simulink model "Napdangdi"  (R2016a)
settings: Solver=FixedStepAuto  StartTime=0.0  StopTime=inf  FixedStep=0.04  RelTol=1e-3
InitFcn:
  | ts=0.04;
  | 
  | v = evalin('base', 'deta1');
  | Deta1 = v;
  | v = evalin('base', 'deta2');
  | Deta2 = v;
  | v = evalin('base', 'deta3');
  | Deta3 = v;
  | v = evalin('base', 'deta5');
  | Deta5 = v;
  | v = evalin('base', 'deta6');
  | Deta6 = v;
  | v = evalin('base', 'deta7');
  | Deta7 = v;
  | v = evalin('base', 'deta8');
  | Deta8 = v;
  | v = evalin('base', 'deta10');
  | Deta10 = v;
  | v = evalin('base', 'deta11');
  | Deta11 = v;
  | v = evalin('base', 'deta12');
  | Deta12 = v;
values from neighbouring files (symbols this model uses):
  deta1 = atan(l.y./l.z)    [biped_backward.m]    (also in dang1.mat = [-0.00346399618455 -0.00193508096073 0.00231722618874 0.0086; dang3.mat = [-0.00346399618455 -0.00185781856517 0.00257715248671 0.0091; dang4.mat = [-0.00346399618455 -0.000867212023118 0.00606051163541 0.015; inverse_kinematic.m = atan(y_l/z_l))
  deta10 = pi-detaC    [biped_backward.m]    (also in inverse_kinematic.m; inverse_kinematics.m)
  deta11 = (deta10-deta8)    [biped_backward.m]    (also in inverse_kinematic.m = (deta10 - deta8); inverse_kinematics.m = deta10-deta8)
  deta12 = atan(r.y./r.z)    [biped_backward.m]    (also in inverse_kinematic.m = atan(y_r/z_r); inverse_kinematics.m)
  deta2 = (deta3-deta5)    [biped_backward.m]    (also in inverse_kinematic.m = (deta3 - deta5); inverse_kinematics.m)
  deta3 = pi-detaA    [biped_backward.m]    (also in inverse_kinematic.m; inverse_kinematics.m)
  deta5 = pi/2 - detaA + detaB + asin(l.x./l_l)    [biped_backward.m]    (also in inverse_kinematic.m = pi/2 - detaA + detaB + asin(x_l/l_l); inverse_kinematics.m)
  deta7 = deta12    [biped_backward.m]    (also in inverse_kinematic.m; inverse_kinematics.m)
  deta8 = pi/2 - detaC + detaD + asin(r.x./l_r)    [biped_backward.m]    (also in inverse_kinematic.m = pi/2 - detaC + detaD + asin(x_r/l_r); inverse_kinematics.m = pi/2 - detaC + detad + asin(r.x./l_r))
libraries: arduinolib x10
settings Model: SimulationMode=external  ExtModeTrigDuration=2  Creator=ACER  LastModifiedBy=ACER
settings OptimizationCC: OptimizeModelRefInitCode=on  LifeSpan=Inf  MaxStackSize=64
settings HardwareCC: ProdBitPerPointer=32  ProdLargestAtomicInteger=Long  ProdLargestAtomicFloat=Double  ProdWordSize=32  ProdHWDeviceType=ARM Compatible->ARM Cortex
settings RTWCC: SystemTargetFile=ert.tlc  HardwareBoard=Arduino Due  TemplateMakefile=ert_default_tmf  GenerateReport=on  Toolchain=Arduino ARM v1.6.1  BuildConfiguration=Faster Runs  IncludeHyperlinkInReport=on  LaunchReport=on  GenerateTraceInfo=on  GenerateTraceReport=on  GenerateTraceReportSl=on  GenerateTraceReportSf=on  GenerateTraceReportEml=on
settings CodeAppCC: ForceParamTrailComments=on  IgnoreCustomStorageClasses=off  OperatorAnnotations=on  SimulinkDataObjDesc=on  SFDataObjDesc=on  MATLABFcnDesc=on  InsertBlockDesc=on  MATLABSourceComments=on
settings ERTTargetCC: SupportContinuousTime=on  SupportVariableSizeSignals=on

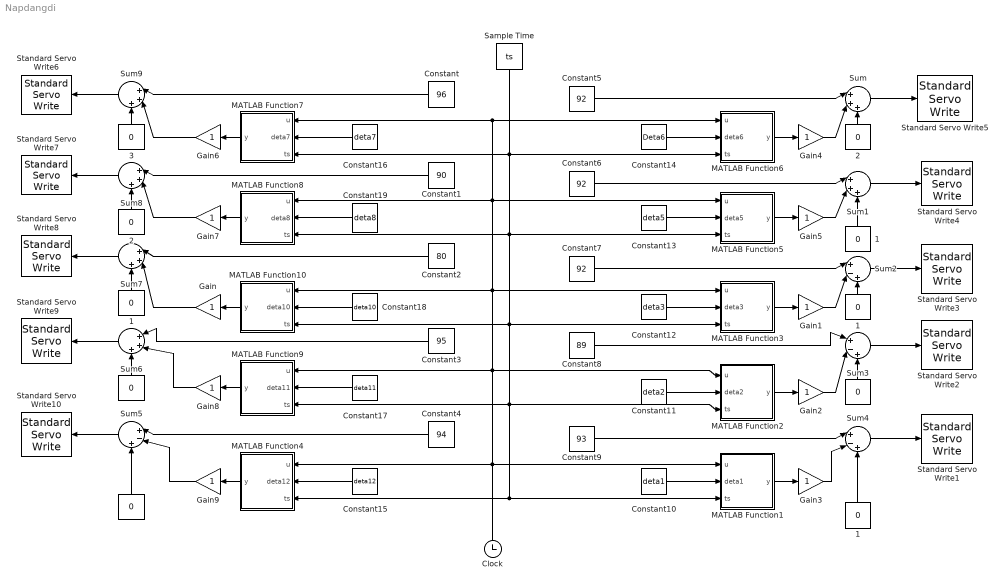
== system Napdangdi ==
   {,,,1,1,1,1..2,2..3} (10 alike) : Constant  Value=0
  Clock : Clock
  Constant : Constant  Value=96
  Constant1 : Constant  Value=90
  Constant10 : Constant  Value=deta1
  Constant11 : Constant  Value=deta2
  Constant12 : Constant  Value=deta3
  Constant13 : Constant  Value=deta5
  Constant14 : Constant  Value=Deta6
  Constant15 : Constant  Value=deta12
  Constant16 : Constant  Value=deta7
  Constant17 : Constant  Value=deta11
  Constant18 : Constant  Value=deta10
  Constant19 : Constant  Value=deta8
  Constant2 : Constant  Value=80
  Constant3 : Constant  Value=95
  Constant4 : Constant  Value=94
  Constant5 : Constant  Value=92
  Constant6 : Constant  Value=92
  Constant7 : Constant  Value=92
  Constant8 : Constant  Value=89
  Constant9 : Constant  Value=93
  Gain{,1..9} (10 alike) : Gain
  MATLAB Function1 : MATLAB Function  TreatAsAtomicUnit=on
  MATLAB Function10 : MATLAB Function  TreatAsAtomicUnit=on
  MATLAB Function2 : MATLAB Function  TreatAsAtomicUnit=on
  MATLAB Function3 : MATLAB Function  TreatAsAtomicUnit=on
  MATLAB Function4 : MATLAB Function  TreatAsAtomicUnit=on
  MATLAB Function5 : MATLAB Function  TreatAsAtomicUnit=on
  MATLAB Function6 : MATLAB Function  TreatAsAtomicUnit=on
  MATLAB Function7 : MATLAB Function  TreatAsAtomicUnit=on
  MATLAB Function8 : MATLAB Function  TreatAsAtomicUnit=on
  MATLAB Function9 : MATLAB Function  TreatAsAtomicUnit=on
  Sample Time : Constant  Value=ts  SampleTime=0.04
  Standard Servo Write1 : arduinolib/Standard Servo Write  pinNumber=2  blockPlatform=arduino
  Standard Servo Write10 : arduinolib/Standard Servo Write  pinNumber=12  blockPlatform=arduino
  Standard Servo Write2 : arduinolib/Standard Servo Write  pinNumber=3  blockPlatform=arduino
  Standard Servo Write3 : arduinolib/Standard Servo Write  pinNumber=4  blockPlatform=arduino
  Standard Servo Write4 : arduinolib/Standard Servo Write  pinNumber=5  blockPlatform=arduino
  Standard Servo Write5 : arduinolib/Standard Servo Write  pinNumber=6  blockPlatform=arduino
  Standard Servo Write6 : arduinolib/Standard Servo Write  pinNumber=8  blockPlatform=arduino
  Standard Servo Write7 : arduinolib/Standard Servo Write  pinNumber=9  blockPlatform=arduino
  Standard Servo Write8 : arduinolib/Standard Servo Write  pinNumber=10  blockPlatform=arduino
  Standard Servo Write9 : arduinolib/Standard Servo Write  pinNumber=11  blockPlatform=arduino
  Sum{,1,6..9} (6 alike) : Sum  Inputs=|+++
  Sum{2..5} (4 alike) : Sum  Inputs=|+-+
  wires:
  Sum/1 -> Standard Servo Write5/1
  Sum1/1 -> Standard Servo Write4/1
  Sum2/1 -> Standard Servo Write3/1
  Sum3/1 -> Standard Servo Write2/1
  Sum4/1 -> Standard Servo Write1/1
  Sum5/1 -> Standard Servo Write10/1
  Sum6/1 -> Standard Servo Write9/1
  Sum7/1 -> Standard Servo Write8/1
  Sum8/1 -> Standard Servo Write7/1
  Sum9/1 -> Standard Servo Write6/1
  MATLAB Function7/1(y) -> Gain6/1
  MATLAB Function8/1(y) -> Gain7/1
  MATLAB Function9/1(y) -> Gain8/1
  MATLAB Function4/1(y) -> Gain9/1
  MATLAB Function2/1(y) -> Gain2/1
  MATLAB Function1/1(y) -> Gain3/1
  MATLAB Function5/1(y) -> Gain5/1
  MATLAB Function6/1(y) -> Gain4/1
  Constant/1 -> Sum9/1
  Constant1/1 -> Sum8/1
  Constant3/1 -> Sum6/1
  Constant4/1 -> Sum5/1
  Constant2/1 -> Sum7/1
  Constant5/1 -> Sum/1
  Constant9/1 -> Sum4/1
  Constant8/1 -> Sum3/1
  Constant7/1 -> Sum2/1
  Constant6/1 -> Sum1/1
  Gain/1 -> Sum7/2
  MATLAB Function10/1(y) -> Gain/1
  MATLAB Function3/1(y) -> Gain1/1
  Gain1/1 -> Sum2/2
  Constant10/1 -> MATLAB Function1/2(deta1)
  Constant11/1 -> MATLAB Function2/2(deta2)
  Constant12/1 -> MATLAB Function3/2(deta3)
  Constant13/1 -> MATLAB Function5/2(deta5)
  Constant14/1 -> MATLAB Function6/2(deta6)
  Constant16/1 -> MATLAB Function7/2(deta7)
  Clock/1 -> MATLAB Function2/1(u), MATLAB Function10/1(u), MATLAB Function5/1(u), MATLAB Function7/1(u), MATLAB Function6/1(u), MATLAB Function8/1(u), MATLAB Function3/1(u), MATLAB Function9/1(u), MATLAB Function4/1(u), MATLAB Function1/1(u)
  Constant17/1 -> MATLAB Function9/2(deta11)
  Constant18/1 -> MATLAB Function10/2(deta10)
  Constant19/1 -> MATLAB Function8/2(deta8)
  Sample Time/1 -> MATLAB Function8/3(ts), MATLAB Function10/3(ts), MATLAB Function3/3(ts), MATLAB Function4/3(ts), MATLAB Function1/3(ts), MATLAB Function2/3(ts), MATLAB Function9/3(ts), MATLAB Function5/3(ts), MATLAB Function7/3(ts), MATLAB Function6/3(ts)
  Gain5/1 -> Sum1/2
  Gain2/1 -> Sum3/2
  Gain3/1 -> Sum4/2
  Gain4/1 -> Sum/2
  Gain6/1 -> Sum9/2
  Gain7/1 -> Sum8/2
  Gain8/1 -> Sum6/2
  Gain9/1 -> Sum5/2
  " "/1 -> Sum5/3
  " "/1 -> Sum3/3
  " "/1 -> Sum6/3
  " 1"/1 -> Sum1/3
  " 1"/1 -> Sum4/3
  " 1"/1 -> Sum7/3
  " 1"/1 -> Sum2/3
  " 2"/1 -> Sum8/3
  " 3"/1 -> Sum9/3
  " 2"/1 -> Sum/3
  Constant15/1 -> MATLAB Function4/2(deta12)

== matlab function Napdangdi/MATLAB Function2 ==
  data: u input; y output; deta2 input; ts input
function y = fcn(u,deta2,ts)
%#codegen
Deta2 = deta2*180/pi;
k = mod(round(u/ts), 201)+1;
y=Deta2(k);

== matlab function Napdangdi/MATLAB Function1 ==
  data: u input; y output; deta1 input; ts input
function y = fcn(u,deta1,ts)
%#codegen
Deta1 = deta1*180/pi;
k = mod(round(u/ts), 201)+1;  
y = Deta1(k);

== matlab function Napdangdi/MATLAB Function3 ==
  data: u input; y output; deta3 input; ts input
function y = fcn(u,deta3,ts)
%#codegen
Deta3 = deta3*180/pi;
k = mod(round(u/ts), 201)+1;
y=Deta3(k);

== matlab function Napdangdi/MATLAB Function5 ==
  data: u input; y output; deta5 input; ts input
function y = fcn(u,deta5,ts)
%#codegen
Deta5 = deta5*180/pi;
k = mod(round(u/ts), 201)+1;
y=Deta5(k);

== matlab function Napdangdi/MATLAB Function6 ==
  data: u input; y output; deta6 input; ts input
function y = fcn(u,deta6,ts)
%#codegen
Deta6 = deta6*180/pi;
k = mod(round(u/ts), 201)+1;
y=Deta6(k);

== matlab function Napdangdi/MATLAB Function7 ==
  data: u input; y output; deta7 input; ts input
function y = fcn(u,deta7,ts)
%#codegen 
Deta7 = deta7*180/pi;    
k = mod(round(u/ts), 201)+1;
y=Deta7(k);

== matlab function Napdangdi/MATLAB Function8 ==
  data: u input; y output; deta8 input; ts input
function y = fcn(u,deta8,ts)
%#codegen
Deta8 = deta8*180/pi;
k = mod(round(u/ts),201)+1;
y=Deta8(k);

== matlab function Napdangdi/MATLAB Function10 ==
  data: u input; y output; deta10 input; ts input
function y = fcn(u,deta10,ts)
%#codegen
Deta10 = deta10*180/pi;
k = mod(round(u/ts), 201)+1;
y=Deta10(k);

== matlab function Napdangdi/MATLAB Function9 ==
  data: u input; y output; deta11 input; ts input
function y = fcn(u,deta11,ts)
%#codegen
Deta11 = deta11*180/pi;
k = mod(round(u/ts), 201)+1;
y=Deta11(k);

== matlab function Napdangdi/MATLAB Function4 ==
  data: u input; y output; deta12 input; ts input
function y = fcn(u,deta12,ts)
%#codegen
Deta12 = deta12*180/pi;
k = mod(round(u/ts), 201)+1;  
y = Deta12(k);
